simulink model "ICARO3_orientation_controllo_BIPE"  (R2014a)
settings: Solver=FixedStepDiscrete  SolverMode=MultiTasking  StartTime=0.0  StopTime=inf  FixedStep=0.001  RelTol=1e-3
PreLoadFcn:
  | Icaro_path;
  | 
  | load_param;
  | 
  | %override compute_alloc_inside load_param !!!
  | compute_alloc_esa;
  | 
  | load('mag_calib_sim_HIL.mat');
  | 
  | init_adaptive;
InitFcn:
  | %define fast control loop sample time
  | ST = 0.005;
  | 
  | %define filters
  | s = tf('s');
  | 
  | % Derivator (useful in PID controller)
  | D = 0.01*s/(0.01*s+1);
  | 
  | % LP 2nd order filter
  | LP = 42.88/(3.5*s^2 + 19.6*s + 42.88);
  | 
  | %load new DP position controllers
  | progetto_controllo_pos_v1;
undefined symbols (not defined in the file): DiscIntNeverNeededParam, Earth, G, H, INV_PITCH_RANGE, INV_ROLL_RANGE, INV_THROTTLE_RANGE, INV_YAW_RANGE, PITCH_IDX, PITCH_MID, ROLL_IDX, ROLL_MID, RTOL, THROTTLE_DOWN, THROTTLE_IDX, THROTTLE_LOW_THRES, Ts, WGS84, YAW_IDX, YAW_MID
libraries: simulink x15, GPIO_Lib x3, cstblocks x2, aerolibtransform2 x1, STM32_Config_Lib x1
(part 2 of 5)

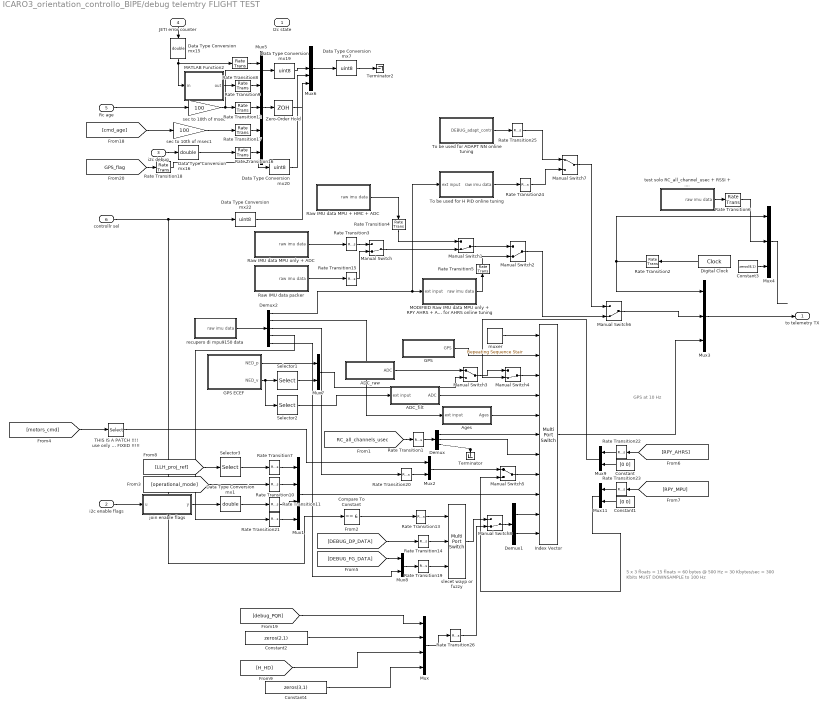
== system ICARO3_orientation_controllo_BIPE/debug telemtry FLIGHT TEST ==
  note: 5 x 3 floats = 15 floats = 60 bytes @ 500 Hz = 30 Kbytes/sec
      | = 300 Kbits
      | MUST DOWNSAMPLE to 100 Hz
  note: GPS at 10 Hz
  I2c state : Inport
  i2c enable flags : Inport  Port=2
  i2c debug : Inport  Port=3
  JETI error counter : Inport  Port=4
  Rc age : Inport  Port=5
  controllr sel : Inport  Port=6
  ADC_filt : Subsystem
  ADC_raw : Subsystem
  Ages : Subsystem
  Compare To Constant : simulink/Logic and Bit Operations/Compare To Constant  relop===  const=6  OutDataTypeStr=uint8
  Constant : Constant  Value=[0 0]  SampleTime=0.01
  Constant1 : Constant  Value=[0 0]  SampleTime=0.01
  Constant2 : Constant  Value=zeros(2,1)  SampleTime=1/400
  Constant3 : Constant  Value=zeros(8,1)  SampleTime=ST
  Constant4 : Constant  Value=zeros(3,1)  SampleTime=1/400
  Data Type Conversion mx1 : DataTypeConversion  OutDataTypeStr=double  RndMeth=Round  SaturateOnIntegerOverflow=on
  Data Type Conversion mx15 : DataTypeConversion  OutDataTypeStr=double  RndMeth=Round  SaturateOnIntegerOverflow=on
  Data Type Conversion mx16 : DataTypeConversion  OutDataTypeStr=double  RndMeth=Round  SaturateOnIntegerOverflow=on
  Data Type Conversion mx{7,19..20,22} (4 alike) : DataTypeConversion  OutDataTypeStr=uint8  RndMeth=Round  SaturateOnIntegerOverflow=on
  Demux : Demux  Outputs=[5 5 2]
  Demux1 : Demux  Outputs=[5 5]
  Demux2 : Demux  Outputs=[1 1 1 1 2]
  Digital Clock : DigitalClock  SampleTime=ST
  GPS : Subsystem
  GPS ECEF : Subsystem
  Index Vector : MultiPortSwitch  DataPortOrder=Zero-based contiguous  Inputs=10  zeroidx=on  SampleTime=0.01
  MATLAB Function2 : MATLAB Function  TreatAsAtomicUnit=on
  MODIFIED Raw IMU data MPU only + RPY AHRS + ALTITUDE (H Hd 0) to be used for AHRS online tuning : Subsystem
  Manual Switch{,1..2,4,6,8} (6 alike) : ManualSwitch  CurrentSetting=0
  Manual Switch3 : ManualSwitch
  Manual Switch5 : ManualSwitch
  Manual Switch7 : ManualSwitch
  Mux : Mux  Inputs=[3 2 2 3]
  Mux1 : Mux  Inputs=[2 1 1 1]
  Mux11 : Mux  Inputs=[3 2]
  Mux2 : Mux  Inputs=[4 1]
  Mux3 : Mux  Inputs=3
  Mux4 : Mux  Inputs=3
  Mux5 : Mux  Inputs=[1 1 1 1 2]
  Mux6 : Mux  Inputs=5
  Mux7 : Mux  Inputs=2
  Mux8 : Mux  Inputs=[8 2]
  Mux9 : Mux  Inputs=[3 2]
  Rate Transition{1,7,10..11,21} (5 alike) : RateTransition  Deterministic=off  OutPortSampleTime=0.01
  Rate Transition{2..6,8..9,12..20,22..26} (21 alike) : RateTransition  Deterministic=off
  Raw IMU data MPU + HMC + ADC : Subsystem
  Raw IMU data MPU only + ADC : Subsystem
  Raw IMU data packer : Subsystem
  Selector1 : Selector  InputPortWidth=3  Indices=[1 2]
  Selector2 : Selector  InputPortWidth=3  Indices=[3]
  Selector3 : Selector  InputPortWidth=3  Indices=[1 2]
  THIS IS A PATCH !!!! use only first 4 motors for canbus TO BE FIXED !!!!! : Selector  InputPortWidth=6  Indices=[1:4]
  Terminator : Terminator
  Terminator2 : Terminator
  To be used for ADAPT NN online tuning : Subsystem
  To be used for H PID online tuning : Subsystem
  Zero-Order Hold : ZeroOrderHold  SampleTime=0.01
  join enable flags : MATLAB Function  TreatAsAtomicUnit=on
  muxer : simulink/Sources/Repeating Sequence Stair  OutValues=[0 1 2 3 4 5 6 7 8 9]  tsamp=0.01  OutMin=[]  OutMax=[]  OutDataTypeStr=double  OutputDataTypeScalingMode=double  OutDataType=fixdt(0,8)  ConRadixGroup=Best Precision: Vector-wise  OutScaling=2^-12
  recupero di mpu9150 data : Subsystem
  sec to 10th of msec : Gain  Gain=100
  sec to 10th of msec1 : Gain  Gain=100
  slecet wayp or fuzzy : MultiPortSwitch  DataPortOrder=Zero-based contiguous  Inputs=2  zeroidx=on  SampleTime=0.01
  test solo RC_all_channel_usec + RSSI + .... : Subsystem
  to telemetry TX : Outport
  wires:
  MATLAB Function2/1(out) -> Rate Transition9/1
  sec to 10th of msec/1 -> Rate Transition12/1, Data Type Conversion mx19/1
  Rate Transition8/1 -> Mux5/1
  Rate Transition9/1 -> Mux5/2
  Data Type Conversion mx15/1 -> MATLAB Function2/1(in), Rate Transition8/1
  Rate Transition12/1 -> Mux5/3
  Data Type Conversion mx16/1 -> Rate Transition16/1
  Rate Transition16/1 -> Mux5/5
  [cmd_age] -> sec to 10th of msec1/1
  sec to 10th of msec1/1 -> Rate Transition17/1
  Rate Transition17/1 -> Mux5/4
  Mux5/1 -> Zero-Order Hold/1
  Data Type Conversion mx19/1 -> Mux6/3
  [GPS_flag] -> Rate Transition18/1
  Mux6/1 -> Data Type Conversion mx7/1
  Data Type Conversion mx20/1 -> Mux6/4
  Rate Transition18/1 -> Data Type Conversion mx20/1
  Data Type Conversion mx22/1 -> Mux6/5
  controllr sel/1 -> Data Type Conversion mx22/1, Compare To Constant/1
  JETI error counter/1 -> Data Type Conversion mx15/1
  Zero-Order Hold/1 -> ?
  Rc age/1 -> sec to 10th of msec/1
  i2c debug/1 -> Data Type Conversion mx16/1
  Raw IMU data packer/1(raw imu data) -> Rate Transition15/1
  Digital Clock/1 -> Rate Transition2/1
  Raw IMU data MPU only + ADC/1(raw imu data) -> Rate Transition3/1
  Rate Transition3/1 -> Manual Switch/1
  Rate Transition15/1 -> Manual Switch/2
  Manual Switch/1 -> Manual Switch1/2
  Raw IMU data MPU + HMC + ADC/1(raw imu data) -> Rate Transition4/1
  Rate Transition4/1 -> Manual Switch1/1
  Manual Switch1/1 -> Manual Switch2/1
  MODIFIED Raw IMU data MPU only + RPY AHRS + ALTITUDE (H Hd 0) to be used for AHRS online tuning/1(raw imu data) -> Rate Transition5/1
  Manual Switch2/1 -> Manual Switch6/2
  Rate Transition5/1 -> Manual Switch2/2
  muxer/1 -> Index Vector/1
  GPS/1(GPS) -> Index Vector/2
  ADC_filt/1(ADC) -> Index Vector/4
  Ages/1(Ages) -> Index Vector/5
  [RC_all_channels_usec] -> Rate Transition1/1
  Demux/3 -> Terminator/1
  Demux/1 -> Index Vector/6
  Demux/2 -> Index Vector/7
  Rate Transition2/1 -> Mux3/1, Mux4/1
  [LLH_proj_ref] -> Selector3/1
  Selector3/1 -> Rate Transition7/1
  Rate Transition1/1 -> Demux/1
  [DEBUG_DP_DATA] -> Rate Transition14/1
  Demux1/1 -> Index Vector/10
  Demux1/2 -> Index Vector/11
  [operational_mode] -> Rate Transition10/1
  Mux1/1 -> Index Vector/9
  i2c enable flags/1 -> join enable flags/1(u)
  join enable flags/1(y) -> Data Type Conversion mx1/1
  Data Type Conversion mx1/1 -> Rate Transition11/1
  Demux2/4 -> Rate Transition21/1
  [motors_cmd] -> THIS IS A PATCH !!!! use only first 4 motors for canbus TO BE FIXED !!!!!/1
  Rate Transition7/1 -> Mux1/1
  Rate Transition10/1 -> Mux1/2
  Rate Transition11/1 -> Mux1/3
  test solo RC_all_channel_usec + RSSI + ..../1(raw imu data) -> Rate Transition6/1
  Rate Transition6/1 -> Mux4/2
  ADC_raw/1(ADC) -> Manual Switch3/1
  Mux7/1 -> Manual Switch3/2
  GPS ECEF/1(NED_p) -> Mux7/1
  GPS ECEF/2(NED_v) -> Selector1/1, Selector2/1
  Selector1/1 -> Mux7/2
  Selector2/1 -> ADC_filt/1(ext input)
  Rate Transition14/1 -> slecet wayp or fuzzy/2
  slecet wayp or fuzzy/1 -> Manual Switch8/1
  Mux8/1 -> Rate Transition19/1
  [DEBUG_FG_DATA] -> Mux8/1
  Compare To Constant/1 -> Rate Transition13/1
  Rate Transition13/1 -> slecet wayp or fuzzy/1
  Rate Transition19/1 -> slecet wayp or fuzzy/3
  recupero di mpu9150 data/1(raw imu data) -> Demux2/1
  Demux2/1 -> MODIFIED Raw IMU data MPU only + RPY AHRS + ALTITUDE (H Hd 0) to be used for AHRS online tuning/1(ext input), To be used for H PID online tuning/1(ext input)
  Demux2/2 -> Ages/1(ext input)
  Demux2/3 -> Rate Transition20/1
  Demux2/5 -> Mux8/2
  Rate Transition20/1 -> Mux2/2
  Rate Transition21/1 -> Mux1/4
  Manual Switch4/1 -> Index Vector/3
  Manual Switch3/1 -> Manual Switch4/1
  Rate Transition22/1 -> Mux9/1
  [RPY_AHRS] -> Rate Transition22/1
  Manual Switch5/1 -> Index Vector/8
  Mux2/1 -> Manual Switch5/1
  Rate Transition23/1 -> Mux11/1
  [RPY_MPU] -> Rate Transition23/1
  Data Type Conversion mx7/1 -> Terminator2/1
  Constant/1 -> Mux9/2
  Constant1/1 -> Mux11/2
  Constant3/1 -> Mux4/3
  Mux3/1 -> to telemetry TX/1
  Mux4/1 -> ?
  Mux9/1 -> Manual Switch4/2
  Mux11/1 -> Manual Switch5/2
  Manual Switch6/1 -> Mux3/2
  To be used for H PID online tuning/1(raw imu data) -> Rate Transition24/1
  Manual Switch7/1 -> Manual Switch6/1
  Rate Transition24/1 -> Manual Switch7/2
  Rate Transition25/1 -> Manual Switch7/1
  To be used for ADAPT NN online tuning/1(DEBUG_adapt_contr) -> Rate Transition25/1
  Manual Switch8/1 -> Demux1/1
  [debug_PQR] -> Mux/1
  Mux/1 -> Rate Transition26/1
  Constant2/1 -> Mux/2
  Rate Transition26/1 -> Manual Switch8/2
  [H_HD] -> Mux/3
  Constant4/1 -> Mux/4
  Index Vector/1 -> Mux3/3
  THIS IS A PATCH !!!! use only first 4 motors for canbus TO BE FIXED !!!!!/1 -> Mux2/1

== system ICARO3_orientation_controllo_BIPE/debug telemtry FLIGHT TEST1 ==
  note: 3
  Digital Clock : DigitalClock  SampleTime=ST
  MODIFIED Raw IMU data MPU only + RPY AHRS + ALTITUDE (H Hd 0) to be used for AHRS online tuning : Subsystem
  Mux : Mux  Inputs=2
  Mux3 : Mux
  Rate Transition1 : RateTransition  Deterministic=off
  Rate Transition2 : RateTransition  Deterministic=off
  Rate Transition5 : RateTransition  Deterministic=off
  Selector : Selector  InputPortWidth=6  Indices=[1:3]
  to telemetry TX : Outport
  wires:
  Rate Transition5/1 -> Mux3/2
  Mux3/1 -> to telemetry TX/1
  Digital Clock/1 -> Rate Transition1/1
  MODIFIED Raw IMU data MPU only + RPY AHRS + ALTITUDE (H Hd 0) to be used for AHRS online tuning/1(raw imu data) -> Rate Transition5/1
  [ArUco_data] -> Selector/1
  [ArUco_flag] -> Mux/2
  Mux/1 -> Mux3/4
  [x_est] -> Rate Transition2/1
  Rate Transition1/1 -> Mux3/1
  Selector/1 -> Mux/1
  Rate Transition2/1 -> Mux3/3

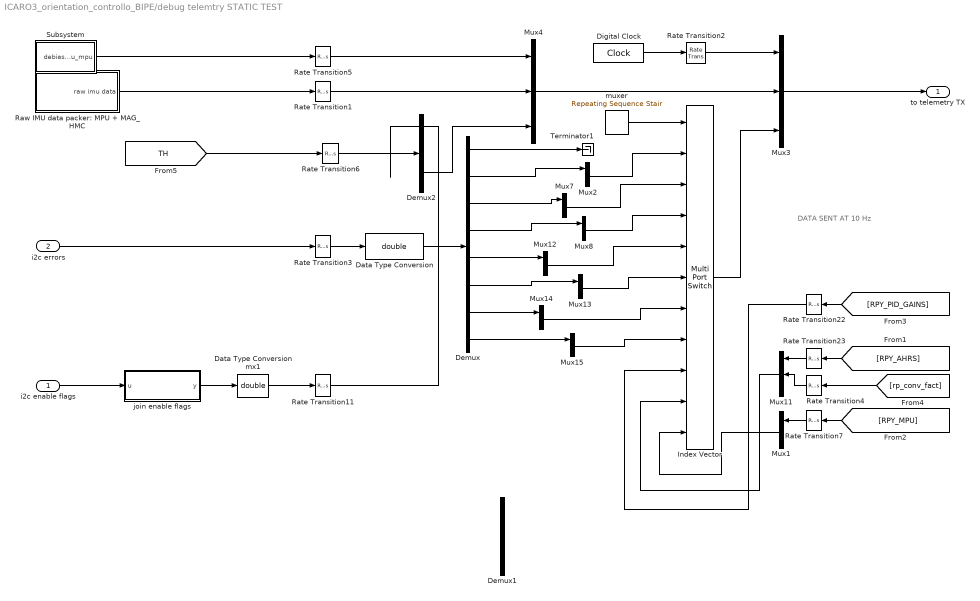
== system ICARO3_orientation_controllo_BIPE/debug telemtry STATIC TEST ==
  note: DATA SENT AT 10 Hz
  i2c enable flags : Inport
  i2c errors : Inport  Port=2
  Data Type Conversion : DataTypeConversion  OutDataTypeStr=double
  Data Type Conversion mx1 : DataTypeConversion  OutDataTypeStr=double  RndMeth=Round  SaturateOnIntegerOverflow=on
  Demux : Demux  Outputs="[2 1 1 1 1 1  1 1]"
  Demux1 : Demux  Outputs=2
  Demux2 : Demux  Outputs=2
  Digital Clock : DigitalClock  SampleTime=ST
  Index Vector : MultiPortSwitch  DataPortOrder=Zero-based contiguous  Inputs=10  zeroidx=on  SampleTime=0.01
  Mux1 : Mux  Inputs=[3 2]
  Mux11 : Mux  Inputs=[3 1 1]
  Mux{2,7..8,12..15} (7 alike) : Mux  Inputs=[1 4]
  Mux3 : Mux  Inputs=3
  Mux4 : Mux  Inputs=3
  Rate Transition{1..2,4..7,22..23} (8 alike) : RateTransition  Deterministic=off
  Rate Transition11 : RateTransition  Deterministic=off  OutPortSampleTime=0.01
  Rate Transition3 : RateTransition  Deterministic=off  OutPortSampleTime=0.01
  Raw IMU data packer: MPU + MAG_HMC : Subsystem
  Subsystem : Subsystem
  Terminator1 : Terminator
  join enable flags : MATLAB Function  TreatAsAtomicUnit=on
  muxer : simulink/Sources/Repeating Sequence Stair  OutValues=[0 1 2 3 4 5 6 7 8 9]  tsamp=0.01  OutMin=[]  OutMax=[]  OutDataTypeStr=double  OutputDataTypeScalingMode=double  OutDataType=fixdt(0,8)  ConRadixGroup=Best Precision: Vector-wise  OutScaling=2^-12
  to telemetry TX : Outport
  wires:
  Rate Transition23/1 -> Mux11/1
  Mux11/1 -> Index Vector/10
  Mux3/1 -> to telemetry TX/1
  Rate Transition11/1 -> ?
  Data Type Conversion mx1/1 -> Rate Transition11/1
  join enable flags/1(y) -> Data Type Conversion mx1/1
  Rate Transition2/1 -> Mux3/1
  Index Vector/1 -> Mux3/3
  muxer/1 -> Index Vector/1
  Digital Clock/1 -> Rate Transition2/1
  i2c enable flags/1 -> join enable flags/1(u)
  Rate Transition7/1 -> Mux1/1
  [RPY_MPU] -> Rate Transition7/1
  Mux1/1 -> Index Vector/11
  Rate Transition22/1 -> Index Vector/9
  i2c errors/1 -> Rate Transition3/1
  Raw IMU data packer: MPU + MAG_HMC/1(raw imu data) -> Rate Transition1/1
  Demux/1 -> Terminator1/1
  Rate Transition3/1 -> Data Type Conversion/1
  Mux4/1 -> Mux3/2
  Data Type Conversion/1 -> Demux/1
  Demux/2 -> Mux2/1
  Demux/3 -> Mux7/1
  Demux/4 -> Mux8/1
  Demux/5 -> Mux12/1
  Demux/6 -> Mux13/1
  Demux/7 -> Mux14/1
  Demux/8 -> Mux15/1
  Mux2/1 -> Index Vector/2
  Mux7/1 -> Index Vector/3
  Mux8/1 -> Index Vector/4
  Mux12/1 -> Index Vector/5
  Mux13/1 -> Index Vector/6
  Mux14/1 -> Index Vector/7
  Mux15/1 -> Index Vector/8
  [RPY_AHRS] -> Rate Transition23/1
  Rate Transition1/1 -> Mux4/2
  [RPY_PID_GAINS] -> Rate Transition22/1
  Rate Transition5/1 -> Mux4/1
  Subsystem/1(debias_imu_mpu) -> Rate Transition5/1
  [rp_conv_fact] -> Rate Transition4/1
  Rate Transition4/1 -> Mux11/2
  [TH] -> Rate Transition6/1
  Demux2/2 -> Mux4/3
  Rate Transition6/1 -> Demux2/1

== matlab function ICARO3_orientation_controllo_BIPE/sensor and actuators interface/interrupt manager/send motor commands via canbus/Subsystem10/MATLAB Function compute gyroxyz1 ==
  settings: updateMethod=DISCRETE  sampleTime=0.01
  data: u input uint16; y output uint8
function y = pack2_8bit(u)

y =uint8([0,0]);
y(1) = bitand(u,255);
y(2) = bitshift(u,-8);

== matlab function ICARO3_orientation_controllo_BIPE/sensor and actuators interface/interrupt manager/send motor commands via canbus/Subsystem10/MATLAB Function compute gyroxyz3 ==
  settings: updateMethod=DISCRETE  sampleTime=0.01
  data: u input uint16; y output uint8
function y = pack2_8bit(u)

y =uint8([0,0]);
y(1) = bitand(u,255);
y(2) = bitshift(u,-8);

== matlab function ICARO3_orientation_controllo_BIPE/sensor and actuators interface/interrupt manager/send motor commands via canbus/Subsystem7/MATLAB Function compute gyroxyz2 ==
  settings: updateMethod=DISCRETE  sampleTime=0.01
  data: u input uint16; y output uint8
function y = pack2_8bit(u)

y =uint8([0,0]);
y(1) = bitand(u,255);
y(2) = bitshift(u,-8);

== matlab function ICARO3_orientation_controllo_BIPE/sensor and actuators interface/interrupt manager/send motor commands via canbus/Subsystem8/MATLAB Function compute gyroxyz1 ==
  settings: updateMethod=DISCRETE  sampleTime=0.01
  data: u input uint16; y output uint8
function y = pack2_8bit(u)

y =uint8([0,0]);
y(1) = bitand(u,255);
y(2) = bitshift(u,-8);

== matlab function ICARO3_orientation_controllo_BIPE/sensor and actuators interface/interrupt manager/send motor commands via canbus/Subsystem8/MATLAB Function compute gyroxyz5 ==
  settings: updateMethod=DISCRETE  sampleTime=0.01
  data: u input uint16; y output uint8
function y = pack2_8bit(u)

y =uint8([0,0]);
y(1) = bitand(u,255);
y(2) = bitshift(u,-8);

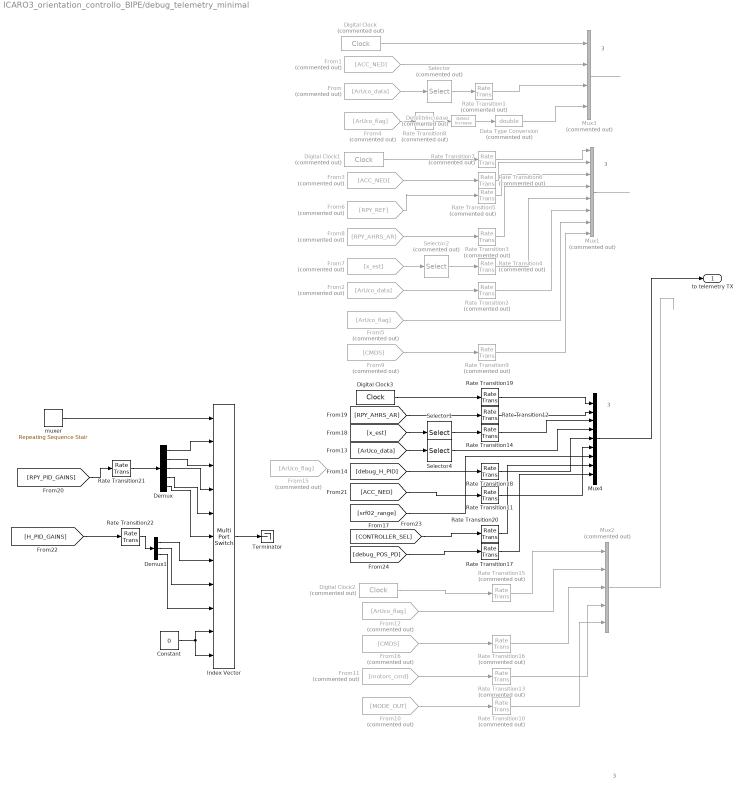
== system ICARO3_orientation_controllo_BIPE/debug_telemetry_minimal ==
  note: 3
  note: 3
  note: 3
  note: 3
  Constant : Constant  Value=0
  Data Type Conversion : DataTypeConversion  Commented=on  OutDataTypeStr=double
  Demux : Demux  Outputs=5
  Demux1 : Demux  Outputs=3
  Detect Increase : simulink/Logic and Bit Operations/Detect Increase  Commented=on  vinit=0.0  InputProcessing=Inherited  OutDataTypeStr=boolean
  Digital Clock : DigitalClock  Commented=on  SampleTime=ST
  Digital Clock1 : DigitalClock  Commented=on  SampleTime=ST
  Digital Clock2 : DigitalClock  Commented=on  SampleTime=ST
  Digital Clock3 : DigitalClock  SampleTime=ST
  From : From  Commented=on  GotoTag=ArUco_data  TagVisibility=global
  From1 : From  Commented=on  GotoTag=ACC_NED  TagVisibility=global
  From10 : From  Commented=on  GotoTag=MODE_OUT  TagVisibility=global
  From11 : From  Commented=on  GotoTag=motors_cmd  TagVisibility=global
  From{4..5,12,15} (4 alike) : From  Commented=on  GotoTag=ArUco_flag  TagVisibility=global
  From16 : From  Commented=on  GotoTag=CMDS  TagVisibility=global
  From2 : From  Commented=on  GotoTag=ArUco_data  TagVisibility=global
  From3 : From  Commented=on  GotoTag=ACC_NED  TagVisibility=global
  From6 : From  Commented=on  GotoTag=RPY_REF
  From7 : From  Commented=on  GotoTag=x_est  TagVisibility=global
  From8 : From  Commented=on  GotoTag=RPY_AHRS_AR  TagVisibility=global
  From9 : From  Commented=on  GotoTag=CMDS  TagVisibility=global
  Index Vector : MultiPortSwitch  DataPortOrder=Zero-based contiguous  Inputs=10  zeroidx=on  SampleTime=0.2
  Mux1 : Mux  Commented=on  Inputs=8
  Mux2 : Mux  Commented=on  Inputs=5
  Mux3 : Mux  Commented=on
  Mux4 : Mux  Inputs=9
  Rate Transition1 : RateTransition  Commented=on  OutPortSampleTime=ST
  Rate Transition{2..7,9..10,13,15..16} (11 alike) : RateTransition  Commented=on
  Rate Transition{11,20..22} (4 alike) : RateTransition  Deterministic=off
  Rate Transition{12,14,17..19} (5 alike) : RateTransition  Deterministic=off  OutPortSampleTime=0.01
  Rate Transition8 : RateTransition  Commented=on  OutPortSampleTime=ST
  Selector : Selector  Commented=on  InputPortWidth=6  Indices=[1:3]
  Selector1 : Selector  InputPortWidth=9  Indices=[4:6]
  Selector2 : Selector  Commented=on  InputPortWidth=9  Indices=[4:6]
  Selector4 : Selector  InputPortWidth=6  Indices=[1:3]
  Terminator : Terminator
  muxer : simulink/Sources/Repeating Sequence Stair  OutValues=[0 1 2 3 4 5 6 7 8 9]  tsamp=0.2  OutMin=[]  OutMax=[]  OutDataTypeStr=double  OutputDataTypeScalingMode=double  OutDataType=fixdt(0,8)  ConRadixGroup=Best Precision: Vector-wise  OutScaling=2^-12
  to telemetry TX : Outport
  wires:
  Selector/1 -> Rate Transition1/1
  Digital Clock/1 -> Mux3/1
  From/1 -> Selector/1
  Mux3/1 -> ?
  From1/1 -> Mux3/2
  Detect Increase/1 -> Data Type Conversion/1
  Rate Transition8/1 -> Detect Increase/1
  From4/1 -> Rate Transition8/1
  Data Type Conversion/1 -> Mux3/4
  Rate Transition1/1 -> Mux3/3
  Digital Clock1/1 -> Rate Transition7/1
  Mux1/1 -> ?
  From3/1 -> Rate Transition6/1
  From5/1 -> Mux1/7
  Rate Transition2/1 -> Mux1/6
  From6/1 -> Rate Transition5/1
  From7/1 -> Selector2/1
  Selector2/1 -> Rate Transition4/1
  Rate Transition4/1 -> Mux1/5
  Rate Transition5/1 -> Mux1/3
  Rate Transition6/1 -> Mux1/2
  Rate Transition7/1 -> Mux1/1
  From8/1 -> Rate Transition3/1
  Rate Transition3/1 -> Mux1/4
  From2/1 -> Rate Transition2/1
  From9/1 -> Rate Transition9/1
  Rate Transition9/1 -> Mux1/8
  Digital Clock2/1 -> Rate Transition15/1
  Mux2/1 -> ?
  From12/1 -> Mux2/2
  Rate Transition15/1 -> Mux2/1
  From16/1 -> Rate Transition16/1
  Rate Transition16/1 -> Mux2/3
  From11/1 -> Rate Transition13/1
  Rate Transition13/1 -> Mux2/4
  From10/1 -> Rate Transition10/1
  Rate Transition10/1 -> Mux2/5
  Digital Clock3/1 -> Rate Transition19/1
  Mux4/1 -> to telemetry TX/1
  [x_est] -> Selector1/1
  Selector1/1 -> Rate Transition14/1
  Rate Transition14/1 -> Mux4/3
  Rate Transition19/1 -> Mux4/1
  [RPY_AHRS_AR] -> Rate Transition12/1
  Rate Transition12/1 -> Mux4/2
  [debug_H_PID] -> Rate Transition18/1
  Rate Transition11/1 -> Mux4/6
  Rate Transition18/1 -> Mux4/5
  [ArUco_data] -> Selector4/1
  Selector4/1 -> Mux4/4
  [ACC_NED] -> Rate Transition11/1
  muxer/1 -> Index Vector/1
  [RPY_PID_GAINS] -> Rate Transition21/1
  Demux/2 -> Index Vector/3
  Demux/3 -> Index Vector/4
  Demux/1 -> Index Vector/2
  Demux/4 -> Index Vector/5
  Demux/5 -> Index Vector/6
  [H_PID_GAINS] -> Rate Transition22/1
  Demux1/1 -> Index Vector/7
  Demux1/2 -> Index Vector/8
  Demux1/3 -> Index Vector/9
  Constant/1 -> Index Vector/10, Index Vector/11
  Index Vector/1 -> Terminator/1
  Rate Transition21/1 -> Demux/1
  Rate Transition22/1 -> Demux1/1
  [srf02_range] -> Mux4/7
  [CONTROLLER_SEL] -> Rate Transition20/1
  [debug_POS_PD] -> Rate Transition17/1
  Rate Transition17/1 -> Mux4/9
  Rate Transition20/1 -> Mux4/8

== system ICARO3_orientation_controllo_BIPE/latch1 ==
  In1 : Inport
  Enable : EnablePort
  Out1 : Outport  InitialOutput=0
  wires:
  In1/1 -> Out1/1

== system ICARO3_orientation_controllo_BIPE/power computations1 ==
  V : Inport
  I : Inport  Port=2
  "1 h in sec " : Constant  Value=3600
  Asec to Ahour : Product  Inputs=*/
  Instantaneous Power : Product  RndMeth=Zero
  integrate current : DiscreteIntegrator  SampleTime=0.01  ICPrevOutput=DiscIntNeverNeededParam  ICPrevScaledInput=DiscIntNeverNeededParam
  low pass filter : cstblocks/LTI System  sys=c2d(tf([10],[1 10]), 0.01)  IC=[]
  low pass filter1 : cstblocks/LTI System  sys=c2d(tf([10],[1 10]), 0.01)  IC=[]
  V_filt : Outport
  I_filt : Outport  Port=2
  P_ist : Outport  Port=3
  I_integ : Outport  Port=4
  wires:
  V/1 -> low pass filter/1
  I/1 -> integrate current/1, low pass filter1/1
  low pass filter/1 -> Instantaneous Power/1, V_filt/1
  low pass filter1/1 -> Instantaneous Power/2, I_filt/1
  Instantaneous Power/1 -> P_ist/1
  integrate current/1 -> Asec to Ahour/1
  Asec to Ahour/1 -> I_integ/1
  "1 h in sec "/1 -> Asec to Ahour/2

== system ICARO3_orientation_controllo_BIPE/pwm & pi cmds ==
  Constant : Constant  Value=[0 0]
  Constant1 : Constant  Value=[0 0]
  Data Type Conversion : DataTypeConversion  OutDataTypeStr=double
  Multiport Switch1 : MultiPortSwitch  DataPortOrder=Zero-based contiguous  Inputs=6
  Multiport Switch2 : MultiPortSwitch  DataPortOrder=Zero-based contiguous  Inputs=6
  mode : Outport
  pi_cmds : Outport  Port=2
  pwm : Outport  Port=3
  wires:
  [mode] -> Multiport Switch1/1, Multiport Switch2/1, Data Type Conversion/1
  Multiport Switch1/1 -> pwm/1
  Constant/1 -> Multiport Switch1/2, Multiport Switch1/3, Multiport Switch1/4, Multiport Switch1/5, Multiport Switch1/6, Multiport Switch1/7
  Multiport Switch2/1 -> pi_cmds/1
  Data Type Conversion/1 -> mode/1
  Constant1/1 -> Multiport Switch2/4, Multiport Switch2/5, Multiport Switch2/7, Multiport Switch2/6, Multiport Switch2/3, Multiport Switch2/2

== system ICARO3_orientation_controllo_BIPE/send gps to bs ==
  note: // gps ecef position
      |     car_telemetry_data.ecef_px = input[0];
      |     car_telemetry_data.ecef_py = input[1];
      |     car_telemetry_data.ecef_pz = input[2];
      |     // gps ecef velocity
      |     car_telemetry_data.ecef_vx = input[3];
      |     car_telemetry_data.ecef_vy = input[4];
      |     car_telemetry_data.ecef_vz = input[5];
      |     // gps_fix
      |     car_telemetry_data.fix = (unsigned char)input[6];
      |     // gps time fix
      |     car_telemetry_data.time_fix = input[7];
      |
      |     // magnetometer data
      |     car_telemetry_data.mag_x = input[8];
      |     car_telemetry_data.mag_y = input[9];
      |     car_telemetry_data.mag_z = input[10];
      |
      |     //execution mode
      |     car_telemetry_data.mode = (unsigned char)input[11];
      |
      |     //pi commands
      |     car_telemetry_data.pi_motore = input[12];
      |     car_telemetry_data.pi_sterzo = input[13];
      |
      |     //pwm commands
      |     car_telemetry_data.pwm_motore = input[14];
      |     car_telemetry_data.pwm_sterzo = input[15];
      |
      |     //heading error
      |     car_telemetry_data.heading_error = input[16];
      |
      |     //input[17]=id_car
  GPS to send : Inport
  MAG to send : Inport  Port=2
  execution mode : Inport  Port=3
  pid_command : Inport  Port=4
  pwm command : Inport  Port=5
  heading_error : Inport  Port=6
  id_car : Inport  Port=7
  Enable : EnablePort
  Mux : Mux  Inputs=7
  S-Function : S-Function  FunctionName=sfun_send_to_bs  EnableBusSupport=off
  wires:
  GPS to send/1 -> Mux/1
  MAG to send/1 -> Mux/2
  Mux/1 -> S-Function/1
  execution mode/1 -> Mux/3
  pid_command/1 -> Mux/4
  pwm command/1 -> Mux/5
  heading_error/1 -> Mux/6
  id_car/1 -> Mux/7

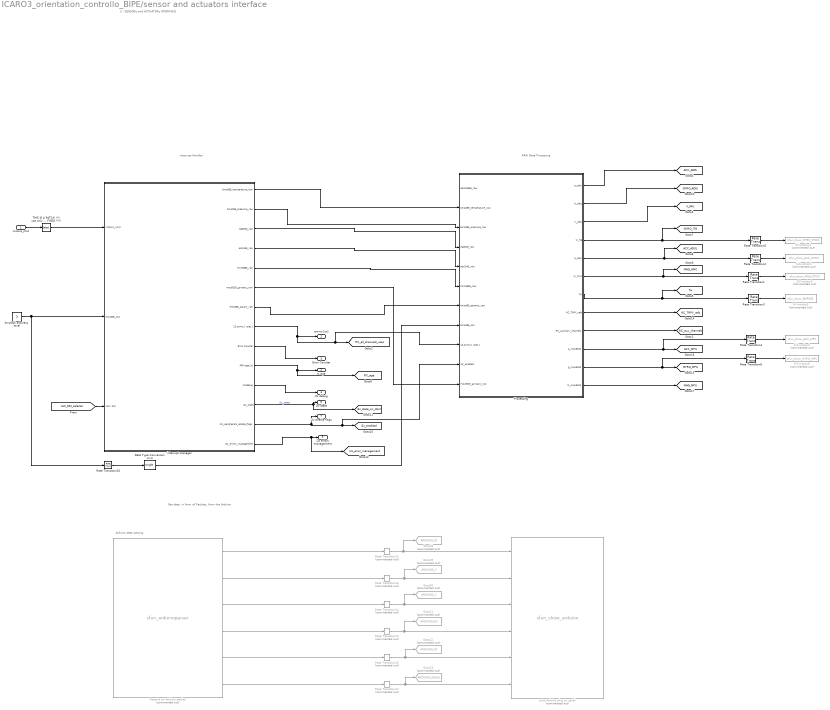
== system ICARO3_orientation_controllo_BIPE/sensor and actuators interface ==
  note: RAW Data Processing
  note: Interrupt Handler
  note: 3 - SENSORs and ACTUATORs INTERFACE
  note: Arduino data parsing
  note: Get data, in form of Packets, from the Arduino
  motors_cmd : Inport
  Data Type Conversion mx3 : DataTypeConversion  OutDataTypeStr=single  RndMeth=Round  SaturateOnIntegerOverflow=on
  Goto18 : Goto  Commented=on  GotoTag=ARDUINO_ID  TagVisibility=global
  Goto19 : Goto  Commented=on  GotoTag=ARDUINO_X  TagVisibility=global
  Goto20 : Goto  Commented=on  GotoTag=ARDUINO_Y  TagVisibility=global
  Goto21 : Goto  Commented=on  GotoTag=ARDUINO_DX  TagVisibility=global
  Goto22 : Goto  Commented=on  GotoTag=ARDUINO_DY  TagVisibility=global
  Goto23 : Goto  Commented=on  GotoTag=ARDUINO_SQUAL  TagVisibility=global
  Processing : Subsystem
  Rate Transition{1..6} (6 alike) : RateTransition
  Rate Transition10 : RateTransition  Deterministic=off
  Rate Transition{12..17} (6 alike) : RateTransition  Commented=on
  Receive an Arduino packet : S-Function  Commented=on  FunctionName=sfun_arduinoparser  Parameters=ST  EnableBusSupport=off
  S-Function1 : S-Function  Commented=on  FunctionName=sfun_show_GYRO_STICK  EnableBusSupport=off
  S-Function2 : S-Function  Commented=on  FunctionName=sfun_show_ACC_STICK  EnableBusSupport=off
  S-Function3 : S-Function  Commented=on  FunctionName=sfun_show_MAG_STICK  EnableBusSupport=off
  S-Function4 : S-Function  Commented=on  FunctionName=sfun_show_ACC_MPU  EnableBusSupport=off
  S-Function5 : S-Function  Commented=on  FunctionName=sfun_show_BMP085  EnableBusSupport=off
  S-Function6 : S-Function  Commented=on  FunctionName=sfun_show_GYRO_MPU  EnableBusSupport=off
  THIS IS A PATCH !!!! use only first 4 motors for canbus TO BE FIXED !!!!! : Selector  InputPortWidth=6  Indices=[1:4]
  bmp085 accuracy level : Constant  Value=3  OutDataTypeStr=uint8
  interrupt manager : Subsystem
  print Arduino pkts on serial : S-Function  Commented=on  FunctionName=sfun_show_arduino  Parameters=ST  EnableBusSupport=off
  pwms [us] : Outport
  rc age : Outport  Port=2
  Error Counter : Outport  Port=3
  i2c debug : Outport  Port=4
  i2c state : Outport  Port=5
  i2c errors management : Outport  Port=6
  i2c enable flags : Outport  Port=7
  tag scope: ACC_ADIS=global, ACC_ADXL=global, ACC_MPU=global, GYRO_ADIS=global, GYRO_ITG=global, GYRO_MPU=global, MAG_HMC=global, MAG_MPU=global, RC_TRPY_refs=global, RC_age=global, RC_all_channels_usec=global, RC_aux_channels=global, TH=global, V_IMU=global, i2c_enabled=global, i2c_error_management=global, i2c_state_on_start=global
  wires:
  Processing/12(m_mpu9150) -> [MAG_MPU]
  Processing/11(g_mpu9150) -> [GYRO_MPU], Rate Transition6/1
  Processing/10(a_mpu9150) -> [ACC_MPU], Rate Transition4/1
  Processing/8(RC_TRPY_refs) -> [RC_TRPY_refs]
  Rate Transition6/1 -> S-Function6/1
  Rate Transition4/1 -> S-Function4/1
  interrupt manager/6(mpu9150_gyroacc_raw) -> Processing/11(mpu9150_gyroacc_raw)
  Processing/4(w_itg) -> Rate Transition5/1, [GYRO_ITG]
  motors_cmd/1 -> THIS IS A PATCH !!!! use only first 4 motors for canbus TO BE FIXED !!!!!/1
  interrupt manager/4(adxl345_raw) -> Processing/5(adxl345_raw)
  Rate Transition5/1 -> S-Function1/1
  Rate Transition3/1 -> S-Function5/1
  Rate Transition2/1 -> S-Function2/1
  Rate Transition1/1 -> S-Function3/1
  [HW_SIM_selector] -> interrupt manager/3(HW / SIM)
  Processing/9(RC_auxiliary_channels) -> [RC_aux_channels]
  interrupt manager/14(i2c_errors_management) -> [i2c_error_management], i2c errors management/1
  interrupt manager/12(i2c_state) -> [i2c_state_on_start], i2c state/1  "i2c_state"
  interrupt manager/11(i2cdebug) -> i2c debug/1
  interrupt manager/9(Error Counter) -> Error Counter/1
  interrupt manager/13(i2c_peripherals_enable_flags) -> Processing/10(i2c_enabled), [i2c_enabled], i2c enable flags/1
  interrupt manager/10(PPM age [s]) -> [RC_age], rc age/1
  interrupt manager/8(12 pwms [ usec ]) -> Processing/9(12 pwms [ usec ]), [RC_all_channels_usec], pwms [us]/1
  Processing/2(w_adis) -> [GYRO_ADIS]
  Processing/1(a_adis) -> [ACC_ADIS]
  Processing/7(TH) -> [TH], Rate Transition3/1
  Processing/5(a_adxl) -> [ACC_ADXL], Rate Transition2/1
  Processing/6(m_hmc) -> Rate Transition1/1, [MAG_HMC]
  Processing/3(V_adis) -> [V_IMU]
  interrupt manager/5(hmc5883_raw) -> Processing/6(hmc5883_raw)
  interrupt manager/1(bmp085_temperature_raw) -> Processing/2(bmp085_temperature_raw)
  interrupt manager/3(itg3200_raw) -> Processing/4(itg3200_raw)
  interrupt manager/2(bmp085_pressure_raw) -> Processing/3(bmp085_pressure_raw)
  interrupt manager/7(bmp085_param_raw) -> Processing/7(bmp085_params_raw)
  Data Type Conversion mx3/1 -> Processing/8(bmp085_oss)
  Rate Transition10/1 -> Data Type Conversion mx3/1
  bmp085 accuracy level/1 -> interrupt manager/2(bmp085_oss), Rate Transition10/1
  THIS IS A PATCH !!!! use only first 4 motors for canbus TO BE FIXED !!!!!/1 -> interrupt manager/1(motors_cmd)
  Receive an Arduino packet/1 -> Rate Transition12/1
  Rate Transition12/1 -> Goto18/1, print Arduino pkts on serial/1
  Receive an Arduino packet/2 -> Rate Transition13/1
  Rate Transition13/1 -> Goto19/1, print Arduino pkts on serial/2
  Receive an Arduino packet/3 -> Rate Transition14/1
  Rate Transition14/1 -> Goto20/1, print Arduino pkts on serial/3
  Receive an Arduino packet/4 -> Rate Transition15/1
  Rate Transition15/1 -> Goto21/1, print Arduino pkts on serial/4
  Receive an Arduino packet/5 -> Rate Transition16/1
  Rate Transition16/1 -> Goto22/1, print Arduino pkts on serial/5
  Receive an Arduino packet/6 -> Rate Transition17/1
  Rate Transition17/1 -> Goto23/1, print Arduino pkts on serial/6

== system ICARO3_orientation_controllo_BIPE/ADIS AHRS2/Attitude Filter ADIS ==
  acc : Inport
  mag : Inport  Port=2
  gyro : Inport  Port=3
  bias : Inport  Port=4
  Enable : EnablePort  StatesWhenEnabling=reset
  DCM_MARG_QUAT : Subsystem  mask{Kp=0.15, Ki=0, tau=40, T=T}
      mask prompts: Kp "Proportional Gain"; Ki "Integral Gain"; tau "Biases Time Constant"; T "Sample Time"
  Data Type Conversion mx3 : DataTypeConversion  OutDataTypeStr=single  RndMeth=Round  SaturateOnIntegerOverflow=on
  Gain1 : Gain  Gain=180/pi
  Rate Transition3 : RateTransition  Deterministic=off
  Scope3 : Scope
      settings: YMin=-140  YMax=80  SaveName=ScopeData14
  Scope4 : Scope
      settings: YMin=-0.08  YMax=0.05  SaveName=ScopeData15
  Scope5 : Scope
      settings: YMin=-4  YMax=4  SaveName=ScopeData16
  Sum : Sum  Inputs=|+-
  Zero-Order Hold2 : ZeroOrderHold  SampleTime=T
  q : Outport  PortDimensions=4  InitialOutput=[1 0 0 0]'
  rpy : Outport  Port=2  PortDimensions=3  InitialOutput=[0 0 0]'
  gyro_bias : Outport  Port=3  PortDimensions=3  InitialOutput=[0 0 0]'
  a_ned : Outport  Port=4  InitialOutput=[0 0 0]'
  wires:
  Gain1/1 -> Scope3/1
  DCM_MARG_QUAT/2(biases) -> Scope4/1, gyro_bias/1
  gyro/1 -> DCM_MARG_QUAT/1(gyro)
  mag/1 -> Rate Transition3/1
  DCM_MARG_QUAT/1(roll_pitch_yaw) -> Gain1/1, rpy/1
  DCM_MARG_QUAT/3(a_ned) -> Scope5/1, a_ned/1
  acc/1 -> Sum/1
  Sum/1 -> Data Type Conversion mx3/1
  DCM_MARG_QUAT/4(q) -> q/1
  Zero-Order Hold2/1 -> DCM_MARG_QUAT/3(mag)
  Rate Transition3/1 -> Zero-Order Hold2/1
  bias/1 -> Sum/2
  Data Type Conversion mx3/1 -> DCM_MARG_QUAT/2(acc)

== system ICARO3_orientation_controllo_BIPE/ADIS AHRS2/debias ADIS ==
  acc : Inport
  gyros : Inport  Port=2
  "Acceleration Detrend " : Subsystem  mask{ST2=ST}
      mask prompts: ST2 "Sample Time"
  Add : Sum  Inputs=+-
  Data Type Conversion mx8 : DataTypeConversion  OutDataTypeStr=single  RndMeth=Round  SaturateOnIntegerOverflow=on
  Gyros Detrend : Subsystem  mask{ST2=ST}
      mask prompts: ST2 "Sample Time"
  Step : Step  SampleTime=ST
  Step1 : Step  Time=11  SampleTime=ST
  acc_out : Outport
  gyro_out : Outport  Port=2
  detrending_ok : Outport  Port=3
  wires:
  Data Type Conversion mx8/1 -> Gyros Detrend/2(Detrending), "Acceleration Detrend "/2(Detrending)
  Gyros Detrend/1(Out) -> gyro_out/1
  "Acceleration Detrend "/1(Out) -> acc_out/1
  gyros/1 -> Gyros Detrend/1(In)
  acc/1 -> "Acceleration Detrend "/1(In)
  Add/1 -> Data Type Conversion mx8/1
  Step1/1 -> detrending_ok/1, Add/2
  Step/1 -> Add/1

== system ICARO3_orientation_controllo_BIPE/ADIS AHRS2/debias ADIS1 ==
  acc : Inport
  gyros : Inport  Port=2
  "Acceleration Detrend " : Subsystem  mask{ST2=ST}
      mask prompts: ST2 "Sample Time"
  Acceleration Detrend 1 : Subsystem  Commented=on  mask{ST2=ST}
      mask prompts: ST2 "Sample Time"
  Add : Sum  Inputs=+-
  Data Type Conversion mx1 : DataTypeConversion  OutDataTypeStr=single  RndMeth=Round  SaturateOnIntegerOverflow=on
  Gyros Detrend : Subsystem  mask{ST2=ST}
      mask prompts: ST2 "Sample Time"
  Step : Step  SampleTime=ST
  Step1 : Step  Time=11  SampleTime=ST
  acc_out : Outport
  gyro_out : Outport  Port=2
  detrending_ok : Outport  Port=3
  wires:
  Gyros Detrend/1(Out) -> gyro_out/1
  "Acceleration Detrend "/1(Out) -> acc_out/1
  gyros/1 -> Gyros Detrend/1(In)
  acc/1 -> "Acceleration Detrend "/1(In)
  Step1/1 -> detrending_ok/1, Add/2
  Step/1 -> Add/1
  Add/1 -> Data Type Conversion mx1/1
  Data Type Conversion mx1/1 -> "Acceleration Detrend "/2(Detrending), Gyros Detrend/2(Detrending)

== system ICARO3_orientation_controllo_BIPE/Control /steer_control ==
  note: The output of the controller is the rise time of the motor pwm in us divided
      | by 1000 (multiplied again by 1000 in sfun_PWM_servomotor).
      | The possible values are within [0.7, 2.2] (the saturation value are set in order to
      | meet this requirement):
      | - [1.52, 2.2] -> turn left
      | - [0.7, 1.52] -> turn right
  note: The controller is proportional and acts according to Control Manager output:
      | - Control Manager output = 1 -> proportional controller ON. This happens if ((startstop = 1) and (distance_to_waypoint > threshold))
      | - Control Manager output = 0 -> proportional controller OFF (The car stops). This happens if ((startstop = 0) and (distance_to_waypoint <= threshold))
      | The value of startstop can be set to 0 manually from Matlab GUI
      | The value of threshold is set to 70cm, so the car has reached the waypoint whether it is 70cm (or less) far from the waypoint
  distance_to_waypoint : Inport
  rel_angle : Inport  Port=2
  startstop : Inport  Port=3
  Constant : Constant  Value=0  SampleTime=0.01
  Constant1 : Constant  Value=1.52
  Control Manager : MATLAB Function  TreatAsAtomicUnit=on
  Gain1 : Gain  Gain=1.2
  Saturation : Saturate  UpperLimit=0.7  LowerLimit=-0.7  SampleTime=0.01
  Sum1 : Sum  Inputs=|++
  Switch1 : Switch  Criteria=u2 > Threshold  Threshold=0.5
  "steer " : Outport
  wires:
  Constant1/1 -> Sum1/2
  distance_to_waypoint/1 -> Control Manager/1(distance)
  Sum1/1 -> "steer "/1
  startstop/1 -> Control Manager/2(startstop)
  Control Manager/1(go) -> Switch1/2
  Constant/1 -> Switch1/3
  Switch1/1 -> Saturation/1
  Gain1/1 -> Switch1/1
  Saturation/1 -> Sum1/1
  rel_angle/1 -> Gain1/1

== system ICARO3_orientation_controllo_BIPE/Control /throttle_control  ==
  note: The output of the controller is the rise time of the motor pwm in ms divided
      | by 1000 (multiplied again by 1000 in sfun_PWM_servomotor).
      | The possible values are within [0.7, 2.2] (the saturation values are set in order to
      | keep a low speed and not going backward):
      | - [1.42, 2.2] -> go backward
      | - [0.7, 1.42] -> go forward
  note: The controller is proportional and acts according to Control Manager output:
      | - Control Manager output = 1 -> proportional controller ON. This happens if ((startstop = 1) and (distance_to_waypoint > threshold))
      | - Control Manager output = 0 -> proportional controller OFF (The car stops). This happens if ((startstop = 0) and (distance_to_waypoint <= threshold))
      | The value of startstop can be set to 0 manually from Matlab GUI
      | The value of threshold is set to 70cm, so the car has reached the waypoint whether it is 70cm (or less) far from the waypoint.
      | The controller has an output speed limiter because the motors don't support rapidly varying pwm values inputs
  distance_to_waypoint : Inport
  startstop : Inport  Port=2
  " zero speed value" : Constant  Value=1.42
  Constant : Constant  Value=0  SampleTime=0.01
  Control Manager : MATLAB Function  TreatAsAtomicUnit=on
  Gain1 : Gain  Gain=-0.001
  MATLAB Function : MATLAB Function  TreatAsAtomicUnit=on
  Memory1 : Memory  InheritSampleTime=on
  Saturation1 : Saturate  UpperLimit=0  LowerLimit=-0.15  SampleTime=0.01
  Sum1 : Sum  Inputs=|++
  Switch1 : Switch  Criteria=u2 > Threshold  Threshold=0.5
  thrrottle : Outport
  wires:
  " zero speed value"/1 -> Sum1/2
  distance_to_waypoint/1 -> Control Manager/1(distance), Gain1/1
  Sum1/1 -> thrrottle/1
  startstop/1 -> Control Manager/2(startstop)
  Gain1/1 -> MATLAB Function/2(current_des_control)
  Control Manager/1(go) -> Switch1/2
  Constant/1 -> Switch1/3
  Switch1/1 -> Saturation1/1
  Memory1/1 -> MATLAB Function/1(prev_des_control)
  MATLAB Function/1(control) -> Switch1/1
  Saturation1/1 -> Memory1/1, Sum1/1

== system ICARO3_orientation_controllo_BIPE/GET PPS/clock latch ==
  In : Inport
  Enable : EnablePort
  Out : Outport  InitialOutput=-1000
  wires:
  In/1 -> Out/1

== system ICARO3_orientation_controllo_BIPE/GET PPS/step 2 pulse ==
  step : Inport
  Logical Operator1 : Logic  AllPortsSameDT=off  OutDataTypeStr=boolean
  Logical Operator2 : Logic  Operator=NOT  AllPortsSameDT=off  OutDataTypeStr=boolean
  Unit Delay : UnitDelay  SampleTime=-1
  pulse : Outport
  wires:
  Logical Operator2/1 -> Unit Delay/1
  Unit Delay/1 -> Logical Operator1/2
  Logical Operator1/1 -> pulse/1
  step/1 -> Logical Operator2/1, Logical Operator1/1

== system ICARO3_orientation_controllo_BIPE/GPS receiver/UBLOX LEA 6 GPS ==
  note: GPS_data (index zero-based):
      | 0: ecef_px
      | 1: ecef_py:
      | 2: ecef_pz
      | 3: ecef_vx
      | 4: ecef_vy
      | 5: ecef_vz
      | 6: gps_fix
  note: // 0: lat
      |                         // 1: lon
      |                         // 2: status
      |                         // 3: speed over ground
      |                         // 4: course over ground
      |                         // 5: gps quality indicator
      |                         // 6: number of satellites
      |                         // 7: hdop
      |                         // 8: altitude
      |                         // 9: dgps station id
      |                        // 10: ECEF Position x
      |                         // 11: ECEF Position y
      |                         // 12: ECEF Position z
      |                         // 13: ECEF Velocity x
      |                         // 14: ECEF Velocity y
      |                         // 15: ECEF Velocity z
  Constant : Constant  Value=0
  Constant1 : Constant  Value=0
  Demux : Demux  Outputs=2
  ECEF Position to LLA : aerolibtransform2/ECEF Position to LLA  units=Metric (MKS)  ptype=Earth (WGS84)  F=1/298.257223563  R=6378137
  MAP ublox fix type to standard status : MATLAB Function  TreatAsAtomicUnit=on
  Mux1 : Mux  Inputs=10
  Mux2 : Mux  Inputs=[10 6]
  S-Function3 : S-Function  FunctionName=sfun_gpsparser_UBLOX  EnableBusSupport=off
  Select ECEF pos : Selector  IndexMode=Zero-based  InputPortWidth=7  Indices=[0 1 2]
  "select ECEF pos + vel " : Selector  IndexMode=Zero-based  InputPortWidth=7  Indices=[0 1 2 3 4 5]
  select GPSFIX : Selector  IndexMode=Zero-based  InputPortWidth=7  Indices=6
  GPS data_16 : Outport
  sync_pulse : Outport  Port=2
  wires:
  S-Function3/2 -> sync_pulse/1
  Select ECEF pos/1 -> ECEF Position to LLA/1
  ECEF Position to LLA/1 -> Demux/1
  Demux/1 -> Mux1/1
  Demux/2 -> Mux1/2
  ECEF Position to LLA/2 -> Mux1/9
  Constant/1 -> Mux1/8, Mux1/7, Mux1/6, Mux1/5, Mux1/4
  Constant1/1 -> Mux1/10
  Mux1/1 -> Mux2/1
  S-Function3/1 -> "select ECEF pos + vel "/1, select GPSFIX/1, Select ECEF pos/1
  Mux2/1 -> GPS data_16/1
  select GPSFIX/1 -> MAP ublox fix type to standard status/1(u)
  "select ECEF pos + vel "/1 -> Mux2/2
  MAP ublox fix type to standard status/1(y) -> Mux1/3

== system ICARO3_orientation_controllo_BIPE/GPS receiver/VENUS GPS ==
  S-Function3 : S-Function  FunctionName=sfun_gpsparser  EnableBusSupport=off
  gps_data_16 : Outport
  sync_pulse : Outport  Port=2
  wires:
  S-Function3/2 -> sync_pulse/1
  S-Function3/1 -> gps_data_16/1

== system ICARO3_orientation_controllo_BIPE/GPS receiver/compute 3d age ==
  gps_fix_quality_flag : Inport
  Compare To Constant : simulink/Logic and Bit Operations/Compare To Constant  relop=>=  const=2.0  OutDataTypeStr=boolean
  Digital Clock : DigitalClock  SampleTime=-1
  Sum : Sum  Inputs=|-+
  clock latch : Subsystem  TreatAsAtomicUnit=on
  gps_3d_fix_age : Outport
  wires:
  Sum/1 -> gps_3d_fix_age/1
  clock latch/1(Out) -> Sum/1
  Digital Clock/1 -> Sum/2, clock latch/1(In)
  gps_fix_quality_flag/1 -> Compare To Constant/1
  Compare To Constant/1 -> clock latch/Enable

== system ICARO3_orientation_controllo_BIPE/GPS receiver/compute age ==
  gps_arrived_flag : Inport
  Digital Clock : DigitalClock  SampleTime=-1
  Sum : Sum  Inputs=|-+
  clock latch : Subsystem  TreatAsAtomicUnit=on
  gps_arrived_flag_out : Outport
  gps_arrived_age : Outport  Port=2
  wires:
  gps_arrived_flag/1 -> gps_arrived_flag_out/1, clock latch/Enable
  Digital Clock/1 -> clock latch/1(In), Sum/2
  clock latch/1(Out) -> Sum/1
  Sum/1 -> gps_arrived_age/1

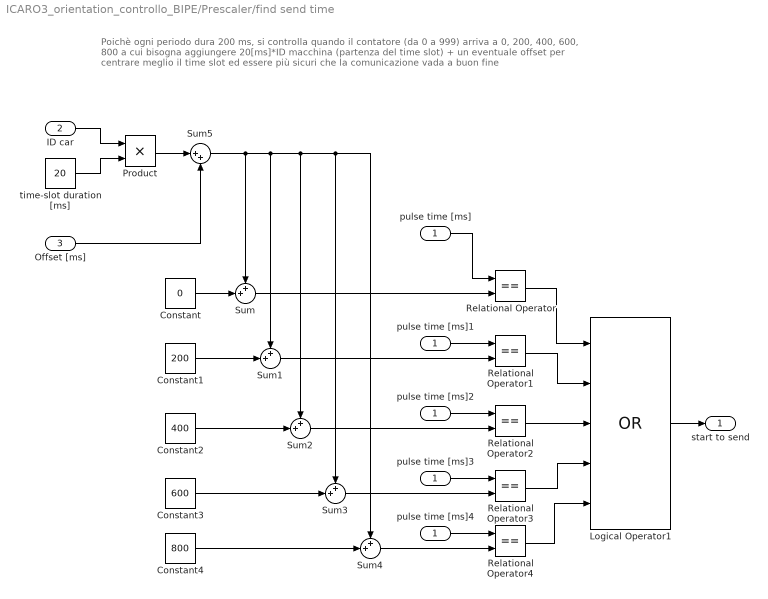
== system ICARO3_orientation_controllo_BIPE/Prescaler/find send time ==
  note: Poichè ogni periodo dura 200 ms,
      | si controlla quando il contatore (da 0 a 999)
      | arriva a 0, 200, 400, 600, 800
      | a cui bisogna aggiungere 20[ms]*ID macchina (partenza del time slot) + un eventuale offset
      | per centrare meglio il time slot ed essere più sicuri che la comunicazione vada a buon fine
  "pulse time [ms] " : Inport
  ID car : Inport  Port=2
  Offset [ms] : Inport  Port=3
  Constant : Constant  Value=0  SampleTime=-1
  Constant1 : Constant  Value=200  SampleTime=-1
  Constant2 : Constant  Value=400  SampleTime=-1
  Constant3 : Constant  Value=600  SampleTime=-1
  Constant4 : Constant  Value=800  SampleTime=-1
  Logical Operator1 : Logic  Operator=OR  Inputs=5  AllPortsSameDT=off  OutDataTypeStr=boolean
  Product : Product
  Relational Operator{,1..4} (5 alike) : RelationalOperator  Operator===  OutDataTypeStr=boolean
  Sum{,1..4} (5 alike) : Sum  Inputs=++|
  Sum5 : Sum  Inputs=|++
  pulse time [ms]{1..4} (4 alike) : InportShadow
  time-slot duration [ms] : Constant  Value=20  SampleTime=-1
  start to send : Outport
  wires:
  ID car/1 -> Product/1
  time-slot duration [ms]/1 -> Product/2
  Constant/1 -> Sum/2
  Sum5/1 -> Sum/1, Sum1/1, Sum2/1, Sum3/1, Sum4/1
  Sum/1 -> Relational Operator/2
  "pulse time [ms] "/1 -> Relational Operator/1
  Constant1/1 -> Sum1/2
  Sum1/1 -> Relational Operator1/2
  pulse time [ms]1/1 -> Relational Operator1/1
  Sum2/1 -> Relational Operator2/2
  pulse time [ms]2/1 -> Relational Operator2/1
  Sum3/1 -> Relational Operator3/2
  pulse time [ms]3/1 -> Relational Operator3/1
  Sum4/1 -> Relational Operator4/2
  pulse time [ms]4/1 -> Relational Operator4/1
  Constant2/1 -> Sum2/2
  Constant3/1 -> Sum3/2
  Constant4/1 -> Sum4/2
  Logical Operator1/1 -> start to send/1
  Relational Operator2/1 -> Logical Operator1/3
  Relational Operator1/1 -> Logical Operator1/2
  Relational Operator/1 -> Logical Operator1/1
  Relational Operator3/1 -> Logical Operator1/4
  Relational Operator4/1 -> Logical Operator1/5
  Offset [ms]/1 -> Sum5/2
  Product/1 -> Sum5/1

== system ICARO3_orientation_controllo_BIPE/Prescaler/latch ==
  In1 : Inport
  Enable : EnablePort
  Out1 : Outport  InitialOutput=[-1000]
  wires:
  In1/1 -> Out1/1

== system ICARO3_orientation_controllo_BIPE/SS AHRS/Attitude Filter SS ==
  acc : Inport
  mag : Inport  Port=2
  gyro : Inport  Port=3
  bias : Inport  Port=4
  Enable : EnablePort  StatesWhenEnabling=reset
  DCM_MARG_QUAT : Subsystem  mask{Kp=0.15, Ki=0, tau=40, T=T}
      mask prompts: Kp "Proportional Gain"; Ki "Integral Gain"; tau "Biases Time Constant"; T "Sample Time"
  Gain1 : Gain  Gain=180/pi
  Rate Transition3 : RateTransition  Deterministic=off
  Scope3 : Scope
      settings: YMin=-140  YMax=80  SaveName=ScopeData14
  Scope4 : Scope
      settings: YMin=-0.08  YMax=0.05  SaveName=ScopeData15
  Scope5 : Scope
      settings: YMin=-4  YMax=4  SaveName=ScopeData16
  Sum : Sum  Inputs=|+-
  Zero-Order Hold2 : ZeroOrderHold  SampleTime=T
  q : Outport  PortDimensions=4  InitialOutput=[1 0 0 0]'
  rpy : Outport  Port=2  PortDimensions=3  InitialOutput=[0 0 0]'
  gyro_bias : Outport  Port=3  PortDimensions=3  InitialOutput=[0 0 0]'
  a_ned : Outport  Port=4  InitialOutput=[0 0 0]'
  wires:
  Rate Transition3/1 -> Zero-Order Hold2/1
  Zero-Order Hold2/1 -> DCM_MARG_QUAT/3(mag)
  DCM_MARG_QUAT/4(q) -> q/1
  bias/1 -> Sum/2
  Sum/1 -> DCM_MARG_QUAT/2(acc)
  acc/1 -> Sum/1
  DCM_MARG_QUAT/3(a_ned) -> a_ned/1, Scope5/1
  DCM_MARG_QUAT/1(roll_pitch_yaw) -> rpy/1, Gain1/1
  mag/1 -> Rate Transition3/1
  gyro/1 -> DCM_MARG_QUAT/1(gyro)
  DCM_MARG_QUAT/2(biases) -> gyro_bias/1, Scope4/1
  Gain1/1 -> Scope3/1

== system ICARO3_orientation_controllo_BIPE/SS AHRS/debias SS ==
  acc : Inport
  gyros : Inport  Port=2
  "Acceleration Detrend " : Subsystem  mask{ST2=ST}
      mask prompts: ST2 "Sample Time"
  Add : Sum  Inputs=+-
  Data Type Conversion mx8 : DataTypeConversion  OutDataTypeStr=single  RndMeth=Round  SaturateOnIntegerOverflow=on
  Gyros Detrend : Subsystem  mask{ST2=ST}
      mask prompts: ST2 "Sample Time"
  Step : Step  SampleTime=ST
  Step1 : Step  Time=11  SampleTime=ST
  acc_out : Outport
  gyro_out : Outport  Port=2
  detrending_ok : Outport  Port=3
  wires:
  Step/1 -> Add/1
  Step1/1 -> Add/2, detrending_ok/1
  Add/1 -> Data Type Conversion mx8/1
  acc/1 -> "Acceleration Detrend "/1(In)
  gyros/1 -> Gyros Detrend/1(In)
  "Acceleration Detrend "/1(Out) -> acc_out/1
  Gyros Detrend/1(Out) -> gyro_out/1
  Data Type Conversion mx8/1 -> "Acceleration Detrend "/2(Detrending), Gyros Detrend/2(Detrending)

== system ICARO3_orientation_controllo_BIPE/blocco motori se non arrivano pacchetti/Enabled Subsystem ==
  In1 : Inport
  Enable : EnablePort
  Out1 : Outport
  wires:
  In1/1 -> Out1/1

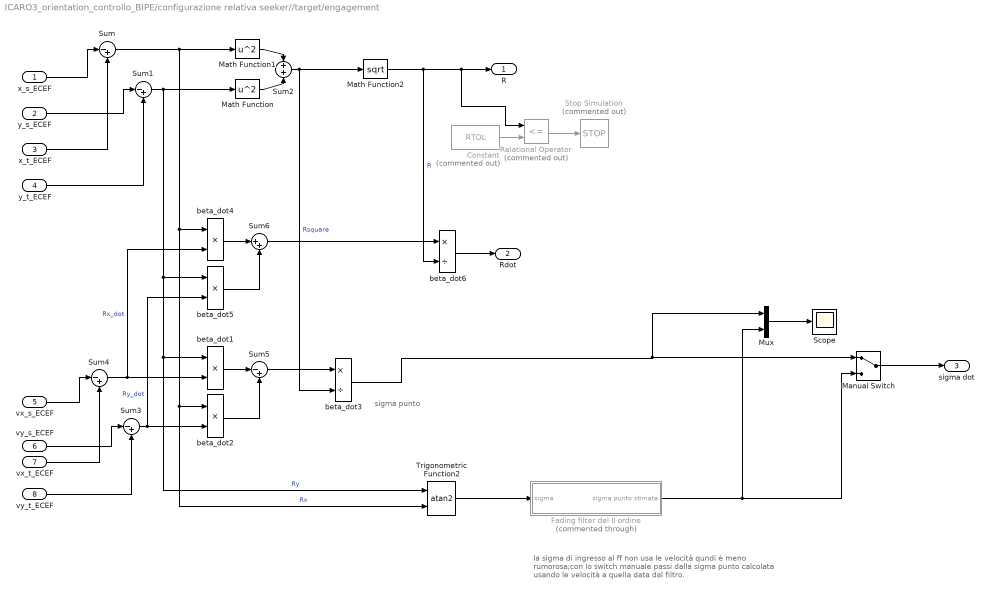
== system ICARO3_orientation_controllo_BIPE/configurazione relativa seeker//target/engagement ==
  note: sigma
      | punto
  note: la sigma di ingresso al ff non usa le velocità qundi
      | è meno rumorosa;con lo switch manuale passi dalla sigma
      | punto calcolata usando le velocità a quella data dal filtro.
  x_s_ECEF : Inport
  y_s_ECEF : Inport  Port=2
  "x_t_ECEF " : Inport  Port=3
  y_t_ECEF : Inport  Port=4
  vx_s_ECEF : Inport  Port=5
  vy_s_ECEF : Inport  Port=6
  vx_t_ECEF : Inport  Port=7
  "vy_t_ECEF " : Inport  Port=8
  Constant : Constant  Commented=on  Value=RTOL
  Fading filter del II ordine : Subsystem  Commented=through
  Manual Switch : ManualSwitch
  Math Function : Math  Operator=square  SaturateOnIntegerOverflow=on
  Math Function1 : Math  Operator=square  SaturateOnIntegerOverflow=on
  Math Function2 : Math  Operator=sqrt  SaturateOnIntegerOverflow=on
  Mux : Mux  Inputs=2
  Relational Operator : RelationalOperator  Commented=on  Operator=<=  OutDataTypeStr=boolean
  Scope : Scope
  Stop Simulation : Stop  Commented=on
  Sum{,1,3..5} (5 alike) : Sum  Inputs=|-+
  Sum2 : Sum  Inputs=+|+
  Sum6 : Sum  Inputs=|++
  Trigonometric Function2 : Trigonometry  Operator=atan2
  beta_dot{1..2,4..5} (4 alike) : Product  Inputs=**
  beta_dot3 : Product  Inputs=*/
  beta_dot6 : Product  Inputs=*/
  R : Outport
  Rdot : Outport  Port=2
  sigma dot : Outport  Port=3
  wires:
  x_s_ECEF/1 -> Sum/1
  "x_t_ECEF "/1 -> Sum/2
  y_s_ECEF/1 -> Sum1/1
  y_t_ECEF/1 -> Sum1/2
  Sum/1 -> Math Function1/1, beta_dot4/1, beta_dot2/1, Trigonometric Function2/2  "Rx"
  Sum1/1 -> Math Function/1, beta_dot5/1, beta_dot1/1, Trigonometric Function2/1  "Ry"
  Math Function1/1 -> Sum2/1
  Math Function/1 -> Sum2/2
  Sum2/1 -> Math Function2/1, beta_dot3/2  "Rsquare"
  Math Function2/1 -> beta_dot6/2, Relational Operator/1, R/1  "R"
  vx_s_ECEF/1 -> Sum4/1
  vx_t_ECEF/1 -> Sum4/2
  vy_s_ECEF/1 -> Sum3/1
  "vy_t_ECEF "/1 -> Sum3/2
  Sum4/1 -> beta_dot1/2, beta_dot4/2  "Rx_dot"
  Sum3/1 -> beta_dot2/2, beta_dot5/2  "Ry_dot"
  beta_dot1/1 -> Sum5/1
  beta_dot2/1 -> Sum5/2
  Sum5/1 -> beta_dot3/1
  beta_dot3/1 -> Mux/1, Manual Switch/1
  beta_dot4/1 -> Sum6/1
  beta_dot5/1 -> Sum6/2
  Sum6/1 -> beta_dot6/1
  Relational Operator/1 -> Stop Simulation/1
  Constant/1 -> Relational Operator/2
  beta_dot6/1 -> Rdot/1
  Fading filter del II ordine/1(sigma punto stimata) -> Manual Switch/2, Mux/2
  Manual Switch/1 -> sigma dot/1
  Trigonometric Function2/1 -> Fading filter del II ordine/1(sigma)
  Mux/1 -> Scope/1

== system ICARO3_orientation_controllo_BIPE/configurazione relativa seeker//target/engagement 2 ==
  Rdot : Inport
  Rdot   to   Vc : Gain  Gain=-1
  Closing Velocity : Outport
  wires:
  Rdot   to   Vc/1 -> Closing Velocity/1
  Rdot/1 -> Rdot   to   Vc/1

== system ICARO3_orientation_controllo_BIPE/configurazione relativa seeker//target/pure PNG  ==
  Closing velocity : Inport
  "sigma dot " : Inport  Port=2
  N : Constant  Value=4
  beta_dot1 : Product  Inputs=**
  beta_dot2 : Product  Inputs=**
  a_c : Outport
  wires:
  Closing velocity/1 -> beta_dot2/1
  beta_dot1/1 -> a_c/1
  "sigma dot "/1 -> beta_dot2/2
  beta_dot2/1 -> beta_dot1/2
  N/1 -> beta_dot1/1

== system ICARO3_orientation_controllo_BIPE/debug telemtry FLIGHT TEST/ADC_filt ==
  ext input : Inport
  Constant : Constant  Value=0
  Mux1 : Mux  Inputs=5
  ADC : Outport
  wires:
  [I_batt_filt] -> Mux1/2
  [V_batt_filt] -> Mux1/1
  [P_batt_filt] -> Mux1/3
  Mux1/1 -> ADC/1
  [I_consumption_Ah] -> Mux1/4
  ext input/1 -> Mux1/5

== system ICARO3_orientation_controllo_BIPE/debug telemtry FLIGHT TEST/ADC_raw ==
  Mux1 : Mux  Inputs=5
  ADC : Outport
  wires:
  Mux1/1 -> ADC/1
  [I_batt] -> Mux1/5
  [V_batt] -> Mux1/4
  [ADC_A2] -> Mux1/3
  [ADC_A0] -> Mux1/1
  [ADC_A1] -> Mux1/2

== system ICARO3_orientation_controllo_BIPE/debug telemtry FLIGHT TEST/Ages ==
  ext input : Inport
  Constant : Constant  Value=0  SampleTime=ST
  Manual Switch2 : ManualSwitch  CurrentSetting=0
  Mux1 : Mux  Inputs=5
  Rate Transition1 : RateTransition  Deterministic=off  OutPortSampleTime=0.01
  Rate Transition4 : RateTransition  Deterministic=off  OutPortSampleTime=0.01
  Rate Transition5 : RateTransition  Deterministic=off  OutPortSampleTime=0.01
  Ages : Outport
  wires:
  [GPS_age] -> Mux1/2
  [GPS_3dfix_age] -> Mux1/1
  [RC_age] -> Rate Transition4/1
  [cmd_age] -> Rate Transition5/1
  Mux1/1 -> Ages/1
  Rate Transition4/1 -> Mux1/3
  Rate Transition5/1 -> Mux1/4
  Constant/1 -> Manual Switch2/1
  ext input/1 -> Manual Switch2/2
  Manual Switch2/1 -> Rate Transition1/1
  Rate Transition1/1 -> Mux1/5
